simulink model "final-sys"  (R2020a)
settings: Solver=VariableStepAuto  StartTime=0.0  StopTime=86400*0.01  RelTol=1e-3
values from neighbouring files (symbols this model uses):
  A = [0              1                   0       0 ... (first row only)    [p4.m]    (also in part3.m)
  B = [ 0             0 ... (first row only)    [p4.m]    (also in part3.m)
  C = [1/r_0      0       0       0 ... (first row only)    [p4.m]    (also in part3.m)
  r_0 = 4.22e7    (= 42200000)    [p4.m]    (also in part3.m)
undefined symbols (not defined in the file or in its folder): ff, K, Knew
settings Model: SimulationMode=accelerator  Creator=mimshin  LastModifiedBy=Edwin

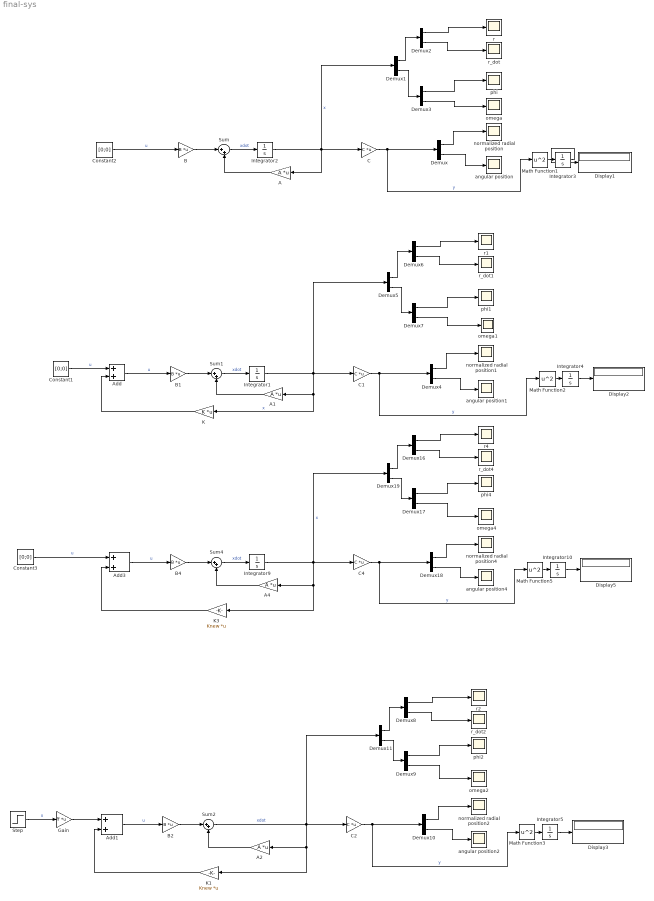
== system final-sys ==
  A{,1..2,4} (4 alike) : Gain  Gain=A  Multiplication=Matrix(K*u)
  Add : Sum
  Add1 : Sum
  Add3 : Sum
  B{,1..2,4} (4 alike) : Gain  Gain=B  Multiplication=Matrix(K*u)
  C{,1..2,4} (4 alike) : Gain  Gain=C  Multiplication=Matrix(K*u)
  Constant1 : Constant  Value=[0;0]  VectorParams1D=off
  Constant2 : Constant  Value=[0;0]  VectorParams1D=off
  Constant3 : Constant  Value=[0;0]  VectorParams1D=off
  Demux{,1..11,16..19} (16 alike) : Demux  Outputs=2
  Display{1..3,5} (4 alike) : Display
  Gain : Gain  Gain=ff  Multiplication=Matrix(K*u)
  Integrator1 : Integrator  InitialCondition=[r_0 0 0 0]'
  Integrator{3..5,10} (4 alike) : Integrator
  Integrator2 : Integrator  InitialCondition=[r_0 0 0 0]'
  Integrator9 : Integrator  InitialCondition=[r_0 0 0 0]'
  K : Gain  Gain=K  Multiplication=Matrix(K*u)
  K1 : Gain  Gain=Knew  Multiplication=Matrix(K*u)
  K3 : Gain  Gain=Knew  Multiplication=Matrix(K*u)
  Math Function{1..3,5} (4 alike) : Math  Operator=square  SignedPower=on  SaturateOnIntegerOverflow=on
  Step : Step  Before=[0; 0];  After=[1; 0];  SampleTime=0
  Sum{,1..2,4} (4 alike) : Sum  Inputs=|++
  angular position{,1..2,4} (4 alike) : Scope
  normalized radial position{,1..2,4} (4 alike) : Scope
  omega{,1..2,4} (4 alike) : Scope
  phi{,1..2,4} (4 alike) : Scope
  r{,1..2,4} (4 alike) : Scope
  r_dot{,1..2,4} (4 alike) : Scope
  wires:
  Constant2/1 -> B/1  "u"
  C/1 -> Demux/1, Math Function1/1  "y"
  Sum/1 -> Integrator2/1  "xdot"
  B/1 -> Sum/1
  A/1 -> Sum/2
  Constant1/1 -> Add/1  "u"
  K/1 -> Add/2
  Math Function1/1 -> Integrator3/1
  Integrator3/1 -> Display1/1
  Demux3/2 -> omega/1
  Demux1/1 -> Demux2/1
  Demux1/2 -> Demux3/1
  Integrator2/1 -> C/1, A/1, Demux1/1  "x"
  Demux2/1 -> r/1
  Demux2/2 -> r_dot/1
  Demux/1 -> normalized radial position/1
  Demux/2 -> angular position/1
  Demux3/1 -> phi/1
  Demux7/1 -> phi1/1
  Demux6/1 -> r1/1
  Demux5/1 -> Demux6/1
  Demux7/2 -> omega1/1
  Demux5/2 -> Demux7/1
  Integrator4/1 -> Display2/1
  B1/1 -> Sum1/1
  Sum1/1 -> Integrator1/1  "xdot"
  Demux6/2 -> r_dot1/1
  C1/1 -> Demux4/1, Math Function2/1  "y"
  A1/1 -> Sum1/2
  Integrator1/1 -> C1/1, K/1, A1/1, Demux5/1  "x"
  Math Function2/1 -> Integrator4/1
  Add/1 -> B1/1  "u"
  Demux4/1 -> normalized radial position1/1
  Demux4/2 -> angular position1/1
  Sum4/1 -> Integrator9/1  "xdot"
  A4/1 -> Sum4/2
  Demux18/2 -> angular position4/1
  Math Function5/1 -> Integrator10/1
  Integrator10/1 -> Display5/1
  Demux17/1 -> phi4/1
  Demux17/2 -> omega4/1
  Demux18/1 -> normalized radial position4/1
  Add3/1 -> B4/1  "u"
  Demux19/2 -> Demux17/1
  Demux16/2 -> r_dot4/1
  B4/1 -> Sum4/1
  Demux19/1 -> Demux16/1
  Demux16/1 -> r4/1
  C4/1 -> Demux18/1, Math Function5/1  "y"
  Integrator9/1 -> C4/1, A4/1, K3/1, Demux19/1  "x"
  K3/1 -> Add3/2
  Constant3/1 -> Add3/1  "u"
  K1/1 -> Add1/2
  Demux9/2 -> omega2/1
  Demux9/1 -> phi2/1
  A2/1 -> Sum2/2
  Sum2/1 -> C2/1, A2/1, K1/1, Demux11/1  "xdot"
  Demux8/1 -> r2/1
  Demux11/2 -> Demux9/1
  Demux10/1 -> normalized radial position2/1
  Integrator5/1 -> Display3/1
  Add1/1 -> B2/1  "u"
  Demux8/2 -> r_dot2/1
  Math Function3/1 -> Integrator5/1
  B2/1 -> Sum2/1
  Demux11/1 -> Demux8/1
  C2/1 -> Demux10/1, Math Function3/1  "y"
  Demux10/2 -> angular position2/1
  Step/1 -> Gain/1  "u"
  Gain/1 -> Add1/1
